simulink model "Simulink1"  (R2025a)
settings: Solver=VariableStepAuto  StartTime=0.0  StopTime=10.0  MaxStep=0.01  RelTol=1e-3
settings Model: Creator=pradipkumarde  LastModifiedBy=pradipkumarde

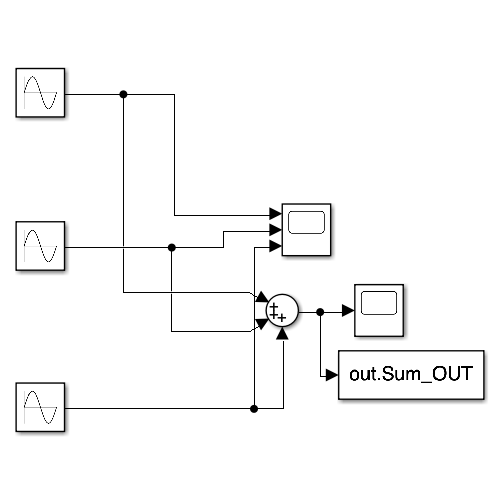
[thumbnail: Simulink's stored preview of the top-level diagram]
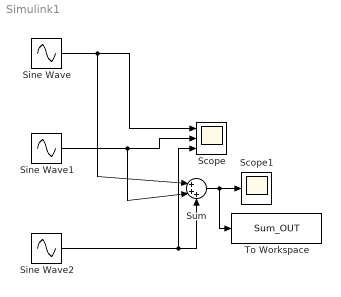
== system Simulink1 ==
  Scope : Scope  NumInputPorts=3
      settings: ActiveDisplayYMinimum=-1.2499967500526621  ActiveDisplayYMaximum=1.2499992865967788
  Scope1 : Scope
      settings: ActiveDisplayYMinimum=-3.4400175950066787  ActiveDisplayYMaximum=3.4399800198065611
  Sine Wave : Sin  SampleTime=0
  Sine Wave1 : Sin  Frequency=5  SampleTime=0
  Sine Wave2 : Sin  Frequency=10  SampleTime=0
  Sum : Sum  Inputs=|+++
  To Workspace : ToWorkspace  VariableName=Sum_OUT  SaveFormat=Timeseries  SampleTime=-1
  wires:
  Sine Wave/1 -> Sum/1, Scope/1
  Sine Wave1/1 -> Sum/2, Scope/2
  Sine Wave2/1 -> Sum/3, Scope/3
  Sum/1 -> To Workspace/1, Scope1/1
